simulink model "alt_nonlinear"  (R2019b)
settings: Solver=VariableStepAuto  StartTime=0.0  StopTime=200  RelTol=1e-3
values from neighbouring files (symbols this model uses):
  Fs = Fl-Fr    [main_rocketmodel.m]    (also in main_sim_rocket.m; rocket_model.m)
  g = 9.8    [main_rocketmodel.m]    (also in main_sim_rocket.m; rocket_model.m; sim_lin.m; test_bangbang.m)
  J_T = 40267    [main_rocketmodel.m]    (also in main_sim_rocket.m; rocket_model.m = 10)
  lower_body = l1+ln    (= 15)    [rocket_model.m]
  m = 549054    [main_rocketmodel.m]    (also in main_sim_rocket.m; rocket_model.m = 25.4; sim_lin.m; test_bangbang.m)
  phi = (1e-6)*square(t_signal,25)    [main_rocketmodel.m]    (also in main_sim_rocket.m = zeros(length(t_signal),1); nominal_trajectory.m = zeros(length(t_signal),1); rocket_model.m = out.phi; sim_lin.m)
  upper_body = l2    (= 3)    [rocket_model.m]
settings Model: Creator=bia  LastModifiedBy=bia
settings DataIOCC: ExternalInput=[t, Fe]  LoadExternalInput=on

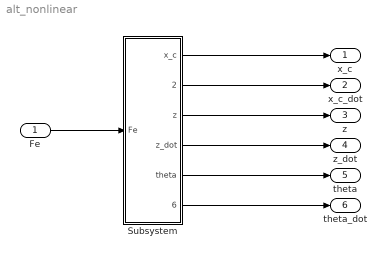
== system alt_nonlinear ==
  Fe : Inport
  Subsystem : Subsystem
  x_c : Outport
  x_c_dot : Outport  Port=2
  z : Outport  Port=3
  "z_dot " : Outport  Port=4
  theta : Outport  Port=5
  "theta_dot " : Outport  Port=6
  wires:
  Fe/1 -> Subsystem/1(Fe)
  Subsystem/1(x_c) -> x_c/1
  Subsystem/2(x_c_dot) -> x_c_dot/1
  Subsystem/3(z) -> z/1
  Subsystem/4("z_dot ") -> "z_dot "/1
  Subsystem/5(theta) -> theta/1
  Subsystem/6("theta_dot ") -> "theta_dot "/1

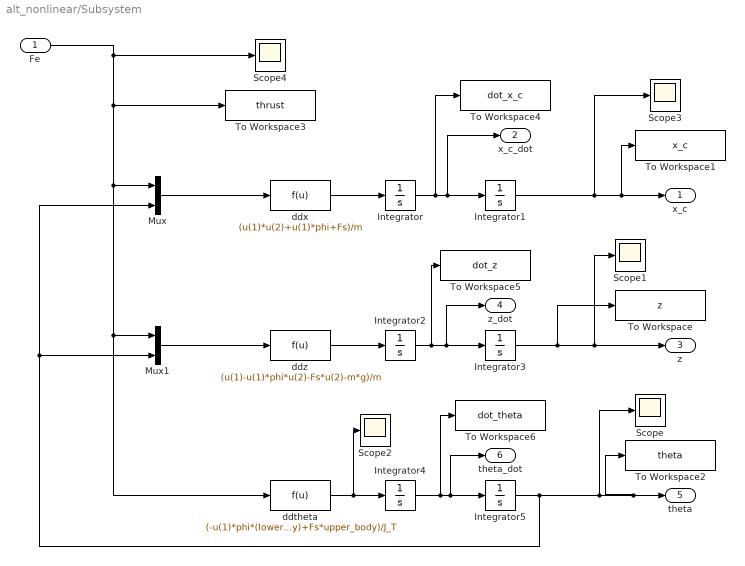
== system alt_nonlinear/Subsystem ==
  Fe : Inport
  Integrator : Integrator  ContinuousStateAttributes='x_c_dot'
  Integrator1 : Integrator  ContinuousStateAttributes='x_c'
  Integrator2 : Integrator  ContinuousStateAttributes='z_dot'
  Integrator3 : Integrator  ContinuousStateAttributes='z'
  Integrator4 : Integrator  ContinuousStateAttributes='theta_dot'
  Integrator5 : Integrator
  Mux : Mux  Inputs=2
  Mux1 : Mux  Inputs=2
  Scope{,1..4} (5 alike) : Scope
  To Workspace : ToWorkspace  VariableName=z  SaveFormat=Timeseries  SampleTime=-1
  To Workspace1 : ToWorkspace  VariableName=x_c  SaveFormat=Timeseries  SampleTime=-1
  To Workspace2 : ToWorkspace  VariableName=theta  SaveFormat=Timeseries  SampleTime=-1
  To Workspace3 : ToWorkspace  VariableName=thrust  SaveFormat=Timeseries  SampleTime=-1
  To Workspace4 : ToWorkspace  VariableName=dot_x_c  SaveFormat=Timeseries  SampleTime=-1
  To Workspace5 : ToWorkspace  VariableName=dot_z  SaveFormat=Timeseries  SampleTime=-1
  To Workspace6 : ToWorkspace  VariableName=dot_theta  SaveFormat=Timeseries  SampleTime=-1
  ddtheta : Fcn  Expr=(-u(1)*phi*(lower_body)+Fs*upper_body)/J_T
  ddx : Fcn  Expr=(u(1)*u(2)+u(1)*phi+Fs)/m
  ddz : Fcn  Expr=(u(1)-u(1)*phi*u(2)-Fs*u(2)-m*g)/m
  x_c : Outport
  x_c_dot : Outport  Port=2
  z : Outport  Port=3
  "z_dot " : Outport  Port=4
  theta : Outport  Port=5
  "theta_dot " : Outport  Port=6
  wires:
  ddx/1 -> Integrator/1
  ddz/1 -> Integrator2/1
  Integrator/1 -> To Workspace4/1, x_c_dot/1, Integrator1/1
  Integrator1/1 -> To Workspace1/1, x_c/1, Scope3/1
  Integrator2/1 -> To Workspace5/1, "z_dot "/1, Integrator3/1
  ddtheta/1 -> Scope2/1, Integrator4/1
  Mux1/1 -> ddz/1
  Integrator4/1 -> To Workspace6/1, Integrator5/1, "theta_dot "/1
  Integrator3/1 -> To Workspace/1, z/1, Scope1/1
  Fe/1 -> Scope4/1, To Workspace3/1, ddtheta/1, Mux1/1, Mux/1
  Mux/1 -> ddx/1
  Integrator5/1 -> Scope/1, To Workspace2/1, theta/1, Mux/2, Mux1/2
